simulink model "mathematicalParameterEstimationTest"  (R2023b)
settings: Solver=VariableStepAuto  StartTime=0.0  StopTime=21600*2  RelTol=1e-3
values from neighbouring files (symbols this model uses):
  C1 = 12.6138    [DPBatteryDynamics.m]    (also in DPBatteryModuleDynamics.m = 174.354594213; MPCControllerForModuleSim.m = 174.354594213; TubeBasedMPCControllerForModuleSim.m = 174.354594213)
  R1 = 3e-4    (= 0.0003)    [DPBatteryDynamics.m]    (also in DPBatteryModuleDynamics.m = 0.00360795873337; MPCControllerForModuleSim.m = 0.00360795873337; TubeBasedMPCControllerForModuleSim.m = 0.00360795873337)
libraries: simulink x1
settings Model: Creator=Adam  LastModifiedBy=Adam

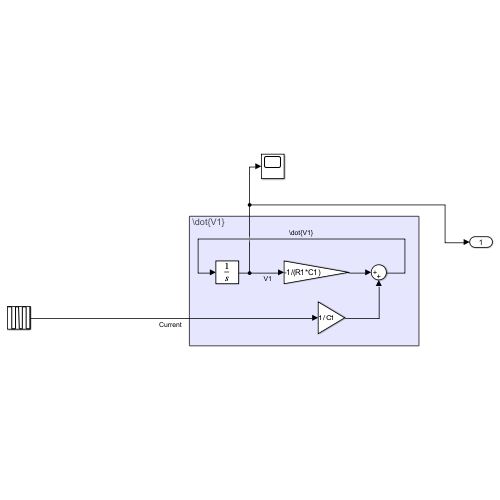
[thumbnail: Simulink's stored preview of the top-level diagram]
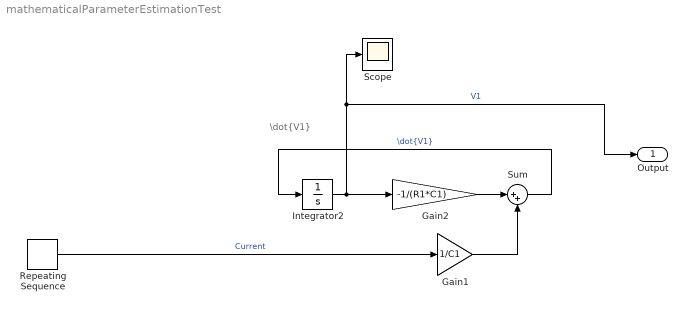
== system mathematicalParameterEstimationTest ==
  note: \dot{V1}
  Gain1 : Gain  Gain=1/C1
  Gain2 : Gain  Gain=-1/(R1*C1)
  Integrator2 : Integrator  InitialCondition=48.95
  Repeating Sequence : simulink/Sources/Repeating Sequence  rep_seq_t=moduleParameterTime  rep_seq_y=moduleParameterCurrent
  Scope : Scope
  Sum : Sum  Inputs=|++
  Output : Outport
  wires:
  Gain1/1 -> Sum/2
  Sum/1 -> Integrator2/1  "\\dot{V1}"
  Gain2/1 -> Sum/1
  Repeating Sequence/1 -> Gain1/1  "Current"
  Integrator2/1 -> Output/1, Scope/1, Gain2/1  "V1"
